simulink model "mmult"  (R2019b)
settings: Solver=VariableStepAuto  StartTime=0.0  StopTime=0  RelTol=1e-3  EnableMultiTasking=on
undefined symbols (not defined in the file): xc7k325tffg900
libraries: ModelComposer x3, simulink x1
settings Model: Creator=dvancamp  LastModifiedBy=viswanad
settings DataIOCC: ReturnWorkspaceOutputs=off
settings OptimizationCC: LifeSpan=inf
settings DebuggingCC: SFUnexpectedBacktrackingDiag=warning  SFNoUnconditionalDefaultTransitionDiag=warning  SFExecutionAtInitializationDiag=none  ArithmeticOperatorsInVariantConditions=warning
settings SFSimCC: SimUseLocalCustomCode=off  CustomCodeUndefinedFunction=UseInterfaceOnly
settings RTWCC: RTWUseLocalCustomCode=off
settings CodeAppCC: StateflowObjectComments=on
settings GRTTargetCC: TargetLangStandard=C89/C90 (ANSI)  GeneratePreprocessorConditionals=Disable all
settings ConfigComp: CovMetricSettings=dw  CovHtmlReporting=on  CovSaveCumulativeToWorkspaceVar=on  CovSaveSingleToWorkspaceVar=on  CovExternalEMLEnable=off

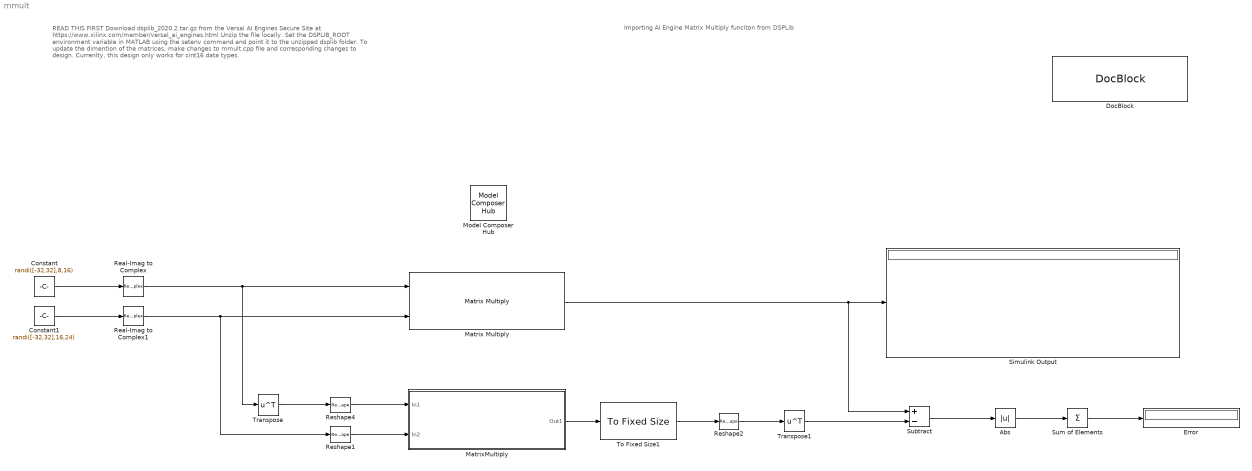
== system mmult ==
  note: READ THIS FIRST
      | Download dsplib_2020.2.tar.gz from the Versal AI Engines Secure Site at https://www.xilinx.com/member/versal_ai_engines.html
      | Unzip the file locally.
      | Set the DSPLIB_ROOT environment variable in MATLAB using the setenv command and point it to the unzipped dsplib folder.
      | To update the dimention of the matrices, make changes to mmult.cpp file and corresponding changes to design.
      | Currenlty, this design only works for cint16 data types.
  note: Importing AI Engine Matrix Multiply funciton from DSPLib
  Abs : Abs
  Constant : Constant  Value=randi([-32,32],8,16)  OutDataTypeStr=int16  SampleTime=1
  Constant1 : Constant  Value=randi([-32,32],16,24)  OutDataTypeStr=int16  SampleTime=1
  DocBlock : simulink/Model-Wide Utilities/DocBlock  DocumentType=Text  mask(DocBlock){}
      content=|
      | ///////////////////////////////////////////////////////////////////////////
      | // Copyright 2020 Xilinx
      | //
      | // Licensed under the Apache License, Version 2.0 (the "License");
      | // you may not use this file except in compliance with the License.
      | // You may obtain a copy of the License at
      | //
      | // http://www.apache.org/licenses/LICENSE-2.0
      | //
      | // Unless required by applicable law or agreed to in writing, software
      | // distributed under the License is distributed on an "AS IS" BASIS,
      | // WITHOUT WARRANTIES OR CONDITIONS OF ANY KIND, either express or implied.
      | // See the License for the specific language governing permissions and
      | // limitations under the License.
      | ///////////////////////////////////////////////////////////////////////////
      mask Display:
      | xmcDrawBlockIcon();
      | disp(['{\fontsize{10pt}(c) Copyright 2020' ' Xilinx, Inc.}\newline \newline '],'texmode','on');
      | disp('{\fontsize{10pt}Licensed under the Apache License 2.0}','texmode','on');
      | disp('\newline \newline \newline{\fontsize{10pt}Double Click for Copyright Notice}','texmode','on');
  Error : Display
  Matrix Multiply : Product  Multiplication=Matrix(*)
  MatrixMultiply : Subsystem
      mask Display: xmcDrawAIEBlockIcon();
  Model Composer Hub : ModelComposer/Model Composer Hub  Description=Performs multiplication  CodeGeneration=off  SubsystemName=MatrixMultiply  TargetDirectory=./code  ExportType=AI Engines  IpVendor=xilinx.com  IpLibrary=hls  IpVersion=1.0  IpHWLanguage=Verilog  AieCompilerOptions={}  CreateTestbench=on  TestbenchStackSize=10  RunAieSim=on  AieSimTimeout=50000  LaunchVitisAnalyzer=off  RunX86Sim=on  X86SimTimeout=10  ProjDevice=Kintex-7 KC705 Evaluation Platform (xc7k325tffg900-2)  ProjDevicePart=xc7k325tffg900-2  SamplePeriod=-1  ClockFrequency=200  DataPathParallelism=1
  Real-Imag to Complex : RealImagToComplex  Input=Real
  Real-Imag to Complex1 : RealImagToComplex  Input=Real
  Reshape1 : Reshape  OutputDimensions=[16,16]
  Reshape2 : Reshape  OutputDimensionality=Customize  OutputDimensions=[24,8]
  Reshape4 : Reshape  OutputDimensions=[16,16]
  Simulink Output : Display
  Subtract : Sum  Inputs=+-  OutDataTypeStr=double
  Sum of Elements : Sum  Inputs=+
  To Fixed Size1 : ModelComposer/To Fixed Size  OutputSize=192  HasStatusOutput=off
  Transpose : Math  Operator=transpose  SignedPower=off  SaturateOnIntegerOverflow=on
  Transpose1 : Math  Operator=transpose  SignedPower=off  SaturateOnIntegerOverflow=on
  wires:
  Constant1/1 -> Real-Imag to Complex1/1
  Constant/1 -> Real-Imag to Complex/1
  Transpose/1 -> Reshape4/1
  To Fixed Size1/1 -> Reshape2/1
  Reshape2/1 -> Transpose1/1
  Transpose1/1 -> Subtract/2
  Matrix Multiply/1 -> Subtract/1, Simulink Output/1
  Subtract/1 -> Abs/1
  Sum of Elements/1 -> Error/1
  Abs/1 -> Sum of Elements/1
  Real-Imag to Complex/1 -> Matrix Multiply/1, Transpose/1
  Real-Imag to Complex1/1 -> Matrix Multiply/2, Reshape1/1
  Reshape4/1 -> MatrixMultiply/1(In1)
  Reshape1/1 -> MatrixMultiply/2(In2)
  MatrixMultiply/1(Out1) -> To Fixed Size1/1

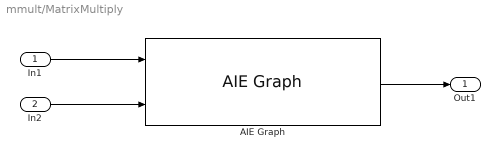
== system mmult/MatrixMultiply ==
  In1 : Inport
  In2 : Inport  Port=2
  AIE Graph : ModelComposer/AIE Graph  PortAttributesTable={ 'Input', 'in1', 'platform.src[0]', 'inA', 'window', 'cint16', '128', 'sync', ''; 'Input', 'in2', 'platform.src[1]', 'inB', 'window', 'cint16', '384', 'sync', ''; 'Output', 'out1', 'platform.sink[0]', 'out', 'window', 'cint16', '192', 'sync', '' }  PortAttributesEnablement={'off', 'off', 'off', 'on', 'off', 'off', 'off', 'off', 'off';'off', 'off', 'off', 'on', 'off', 'off', 'off', 'off', 'off';'off', 'off', 'off', 'on', 'off', 'off', 'off', 'off', 'off'}  PortArgDecls={'in window cint16 in1'; 'in window cint16 in2'; 'out window cint16 out1'}  PortNames={'in1'; 'in2'; 'out1'}  PortAliases={'platform.src[0]'; 'platform.src[1]'; 'platform.sink[0]'}  PortGraphPortNames={'inA'; 'inB'; 'out'}  PortTypes={'window'; 'window'; 'window'}  PortDataTypes={'cint16'; 'cint16'; 'cint16'}  PortSizes={1.280000000000000000e+02; 3.840000000000000000e+02; 1.920000000000000000e+02}  PortSynchronicities={'sync'; 'sync'; 'sync'}  PortSignalSizes={0.000000000000000000e+00; 0.000000000000000000e+00; 0.000000000000000000e+00}  SimLibPath=''  FunctionTabVisible=on  GraphName=xf::dsp::aie::blas::matrix_mult::matrix_mult_graph<cint16, cint16, 8, 16, 24, 0, 0, 0, 1, 0, 128, 384, 1>  GraphHeaderFiles={'/proj/xsjhdstaff4/abehbood/dsplib_2020.2.tar/dsplib/L2/include/hw/matrix_mult_graph.hpp'; '/proj/xsjhdstaff4/abehbood/dsplib_2020.2.tar/dsplib/L1/include/hw/matrix_mult.hpp'}  GraphSourceFile=mmult.cpp  GraphSearchPaths={'$DSPLIB_ROOT/L1/include/hw', '$DSPLIB_ROOT/L2/include/hw', '$DSPLIB_ROOT/L1/src/hw', '$DSPLIB_ROOT/L1/tests/inc'}  GraphPreProcOptions={}
  Out1 : Outport
  wires:
  In2/1 -> AIE Graph/2
  In1/1 -> AIE Graph/1
  AIE Graph/1 -> Out1/1
